simulink model "EXP4"  (R2020b)
settings: Solver=VariableStepAuto  StartTime=0.0  StopTime=0.02  RelTol=1e-3
libraries: powerlib x73, powerlib_meascontrol x2, simulink x2, simulink_extras x1
settings Model: Creator=pushp  LastModifiedBy=rupes
settings DebuggingCC: SFMachineParentedDataDiag=error  ArithmeticOperatorsInVariantConditions=warning
settings SFSimCC: CustomCodeUndefinedFunction=UseInterfaceOnly
settings CodeAppCC: StateflowObjectComments=on

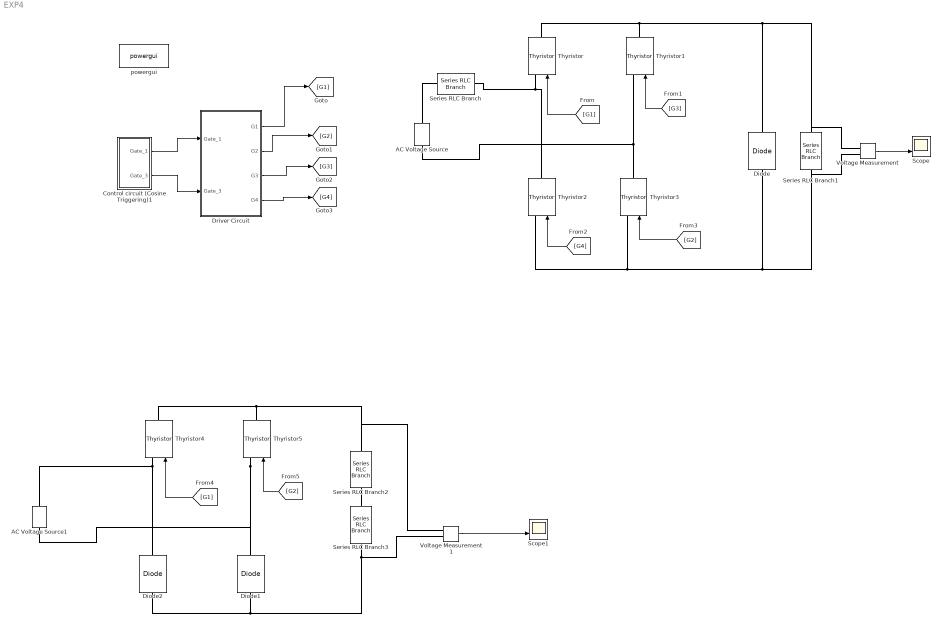
== system EXP4 ==
  AC Voltage Source : powerlib/Electrical Sources/AC Voltage Source  Amplitude=100  Phase=0  Frequency=60  SampleTime=0  Measurements=None  BusType=swing  Pref=10e3  Qref=0  Qmin=-inf  Qmax=+inf
  AC Voltage Source1 : powerlib/Electrical Sources/AC Voltage Source  Amplitude=100  Phase=0  Frequency=60  SampleTime=0  Measurements=None  BusType=swing  Pref=10e3  Qref=0  Qmin=-inf  Qmax=+inf
  Control circuit (Cosine Triggering)1 : Subsystem
  Diode : powerlib/Power Electronics/Diode  Ron=0.001  Lon=0  Vf=0.8  IC=0  UseSnubber=0  Rs=500  Cs=250e-9  Measurements=off
  Diode1 : powerlib/Power Electronics/Diode  Ron=0.001  Lon=0  Vf=0.8  IC=0  UseSnubber=0  Rs=500  Cs=250e-9  Measurements=off
  Diode2 : powerlib/Power Electronics/Diode  Ron=0.001  Lon=0  Vf=0.8  IC=0  UseSnubber=0  Rs=500  Cs=250e-9  Measurements=off
  Driver Circuit : Subsystem
  Scope : Scope  NumInputPorts=2
  Scope1 : Scope  NumInputPorts=2
  Series RLC Branch : powerlib/Elements/Series RLC Branch  LConnTagsString=__new0  RConnTagsString=__new0  BranchType=L  Resistance=1  Inductance=1e-3  SetiL0=off  InitialCurrent=0  Capacitance=1e-6  Setx0=off  InitialVoltage=0  Measurements=None
  Series RLC Branch1 : powerlib/Elements/Series RLC Branch  LConnTagsString=__new0  RConnTagsString=__new0  BranchType=R  Resistance=1  Inductance=1e-3  SetiL0=off  InitialCurrent=0  Capacitance=1e-6  Setx0=off  InitialVoltage=0  Measurements=None
  Series RLC Branch2 : powerlib/Elements/Series RLC Branch  LConnTagsString=__new0  RConnTagsString=__new0  BranchType=L  Resistance=1  Inductance=1e-3  SetiL0=off  InitialCurrent=0  Capacitance=1e-6  Setx0=off  InitialVoltage=0  Measurements=None
  Series RLC Branch3 : powerlib/Elements/Series RLC Branch  LConnTagsString=__new0  RConnTagsString=__new0  BranchType=R  Resistance=1  Inductance=1e-3  SetiL0=off  InitialCurrent=0  Capacitance=1e-6  Setx0=off  InitialVoltage=0  Measurements=None
  Thyristor{,1..5} (6 alike) : powerlib/Power Electronics/Thyristor  Ron=0.001  Lon=0  Vf=0.8  IC=0  Rs=500  Cs=250e-9  Measurements=off
  Voltage Measurement : powerlib/Measurements/Voltage Measurement  PhasorSimulation=off  OutputType=Complex  PSBequivalent=0
  Voltage Measurement1 : powerlib/Measurements/Voltage Measurement  PhasorSimulation=off  OutputType=Complex  PSBequivalent=0
  powergui : powerlib/powergui  Priority=1  SimulationMode=Discrete  SampleTime=1e-6  frequency=60  Iterations=50  frequencyindice=0  Pbase=100e6  ErrMax=1e-4  UnitsV=kV  UnitsW=MW  buscounter=0  FunctionMessages=off  echomessages=off  EnableUseOfTLC=off  CurrentSourceSwitches=off  DisableSnubberDevices=off  DisableRonSwitches=off  DisableVfSwitches=off  DisplayEquations=off  AutomaticDiscreteSolvers=off  SolverType=Tustin/Backward Euler (TBE)  Interpol=off  ExternalGateDelay=off  methode=off  Ts=100  x0status=blocks  SPID=on  SwTol=0  HookPort=off  NonlinearTolerance=1e-4  nMaxIteration=100  ContinueOnMaxIteration=off  RestoreLinks=warning  ResistiveCurrentMeasurement=off  Frange=[0:2:500]  Ylog=off  Xlog=on  ShowGrid=off  save=off  variable=ZData  structure=0  ZoomFFT=off  StartTime=0.0  cycles=1  DisplayStyle=1  fundamental=60  FreqAxis=off  MaxFrequency=1000  frequencyindicesteady=1  RmsSteady=1  display=off
  wires:
  Driver Circuit/4(G4) -> [G4]
  Driver Circuit/1(G1) -> [G1]
  Control circuit (Cosine Triggering)1/1(Gate_1) -> Driver Circuit/1(Gate_1)
  Control circuit (Cosine Triggering)1/2(Gate_3) -> Driver Circuit/2(Gate_3)
  Driver Circuit/3(G3) -> [G3]
  Driver Circuit/2(G2) -> [G2]
  [G1] -> Thyristor/1
  [G3] -> Thyristor1/1
  [G4] -> Thyristor2/1
  [G2] -> Thyristor3/1
  Voltage Measurement/1 -> Scope/2
  [G1] -> Thyristor4/1
  [G2] -> Thyristor5/1
  Voltage Measurement1/1 -> Scope1/2
  connections:
  Thyristor/LConn1 -- Series RLC Branch/RConn1 -- Thyristor2/RConn1
  AC Voltage Source/RConn1 -- Series RLC Branch/LConn1
  Diode/LConn1 -- Voltage Measurement/LConn2 -- Series RLC Branch1/RConn1 -- Thyristor3/LConn1 -- Thyristor2/LConn1
  Thyristor3/RConn1 -- AC Voltage Source/LConn1 -- Thyristor1/LConn1
  Thyristor1/RConn1 -- Thyristor/RConn1 -- Voltage Measurement/LConn1 -- Series RLC Branch1/LConn1 -- Diode/RConn1
  Thyristor5/RConn1 -- Voltage Measurement1/LConn1 -- Series RLC Branch2/LConn1 -- Thyristor4/RConn1
  Series RLC Branch3/RConn1 -- Diode1/LConn1 -- Diode2/LConn1 -- Voltage Measurement1/LConn2
  Thyristor5/LConn1 -- Diode1/RConn1 -- AC Voltage Source1/LConn1
  Thyristor4/LConn1 -- AC Voltage Source1/RConn1 -- Diode2/RConn1
  Series RLC Branch3/LConn1 -- Series RLC Branch2/RConn1

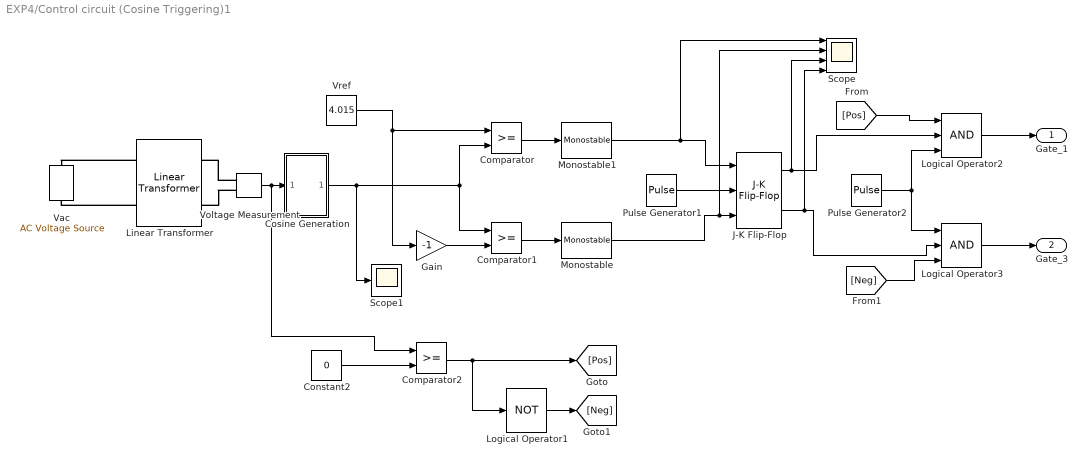
== system EXP4/Control circuit (Cosine Triggering)1 ==
  Comparator : RelationalOperator  OutDataTypeStr=boolean  RndMeth=Nearest
  Comparator1 : RelationalOperator  OutDataTypeStr=boolean  RndMeth=Nearest
  Comparator2 : RelationalOperator  OutDataTypeStr=boolean  RndMeth=Nearest
  Constant2 : Constant  Value=0
  Cosine Generation : Subsystem
  Gain : Gain  Gain=-1
  J-K Flip-Flop : simulink_extras/Flip Flops/J-K Flip-Flop  initial_condition=0
  Linear Transformer : powerlib/Elements/Linear Transformer  UNITS=pu  NominalPower=[4 50 ]  winding1=[230 6.9 7.1e-3 ]  winding2="[3.605 1.7e-3  2.1e-6]"  ThreeWindings=off  winding3=[ 315e3 0.002 0.08 ]  RmLm=[600 1.145]  Measurements=None  DataType=off
  Logical Operator1 : Logic  Operator=NOT  Inputs=inv  IconShape=distinctive  AllPortsSameDT=off  OutDataTypeStr=boolean
  Logical Operator2 : Logic  Inputs=3  IconShape=distinctive  AllPortsSameDT=off  OutDataTypeStr=boolean
  Logical Operator3 : Logic  Inputs=3  IconShape=distinctive  AllPortsSameDT=off  OutDataTypeStr=boolean
  Monostable : powerlib_meascontrol/Logic/Monostable  EdgeDetect=Rising  PulseDuration=1e-05  ic=0  Ts=0
      settings: SourceProductBaseCode=PS
  Monostable1 : powerlib_meascontrol/Logic/Monostable  EdgeDetect=Rising  PulseDuration=1e-05  ic=0  Ts=0
      settings: SourceProductBaseCode=PS
  Pulse Generator1 : DiscretePulseGenerator  PulseType=Time based  Period=2e-5  PulseWidth=50
  Pulse Generator2 : DiscretePulseGenerator  PulseType=Time based  Period=40e-6  PulseWidth=50
  Scope : Scope  NumInputPorts=4
  Scope1 : Scope
  Vac : powerlib/Electrical Sources/AC Voltage Source  Amplitude=230*sqrt(2)  Phase=0  Frequency=50  SampleTime=0  Measurements=None  BusType=swing  Pref=10e3  Qref=0  Qmin=-inf  Qmax=+inf
  Voltage Measurement : powerlib/Measurements/Voltage Measurement  PhasorSimulation=off  OutputType=Complex  PSBequivalent=0
  Vref : Constant  Value=4.015
  Gate_1 : Outport
  Gate_3 : Outport  Port=2
  wires:
  [Neg] -> Logical Operator3/3
  [Pos] -> Logical Operator2/1
  Logical Operator1/1 -> [Neg]
  Comparator2/1 -> [Pos], Logical Operator1/1
  Constant2/1 -> Comparator2/2
  Vref/1 -> Comparator/1, Gain/1
  Logical Operator3/1 -> Gate_3/1
  Logical Operator2/1 -> Gate_1/1
  Pulse Generator2/1 -> Logical Operator3/1, Logical Operator2/3
  J-K Flip-Flop/2 -> Scope/4, Logical Operator3/2
  J-K Flip-Flop/1 -> Logical Operator2/2, Scope/3
  Pulse Generator1/1 -> J-K Flip-Flop/2
  Monostable/1 -> Scope/2, J-K Flip-Flop/3
  Comparator1/1 -> Monostable/1
  Comparator/1 -> Monostable1/1
  Gain/1 -> Comparator1/2
  Cosine Generation/1(Out1) -> Scope1/1, Comparator/2, Comparator1/1
  Voltage Measurement/1 -> Cosine Generation/1(In1), Comparator2/1
  Monostable1/1 -> Scope/1, J-K Flip-Flop/1
  connections:
  Linear Transformer/LConn1 -- Vac/RConn1
  Linear Transformer/LConn2 -- Vac/LConn1
  Voltage Measurement/LConn1 -- Linear Transformer/RConn1
  Voltage Measurement/LConn2 -- Linear Transformer/RConn2

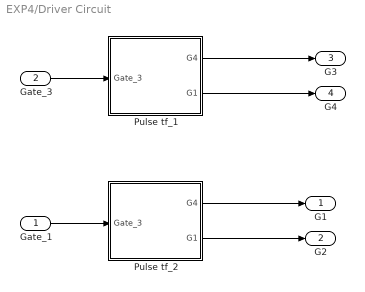
== system EXP4/Driver Circuit ==
  Gate_1 : Inport
  Gate_3 : Inport  Port=2
  Pulse tf_1 : Subsystem
  Pulse tf_2 : Subsystem
  G1 : Outport
  G2 : Outport  Port=2
  G3 : Outport  Port=3
  G4 : Outport  Port=4
  wires:
  Pulse tf_1/1(G4) -> G3/1
  Pulse tf_1/2(G1) -> G4/1
  Gate_3/1 -> Pulse tf_1/1(Gate_3)
  Gate_1/1 -> Pulse tf_2/1(Gate_3)
  Pulse tf_2/1(G4) -> G1/1
  Pulse tf_2/2(G1) -> G2/1

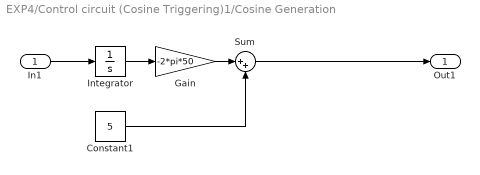
== system EXP4/Control circuit (Cosine Triggering)1/Cosine Generation ==
  In1 : Inport
  Constant1 : Constant  Value=5
  Gain : Gain  Gain=-2*pi*50
  Integrator : Integrator
  Sum : Sum  Inputs=|++
  Out1 : Outport
  wires:
  Sum/1 -> Out1/1
  Constant1/1 -> Sum/2
  In1/1 -> Integrator/1
  Integrator/1 -> Gain/1
  Gain/1 -> Sum/1

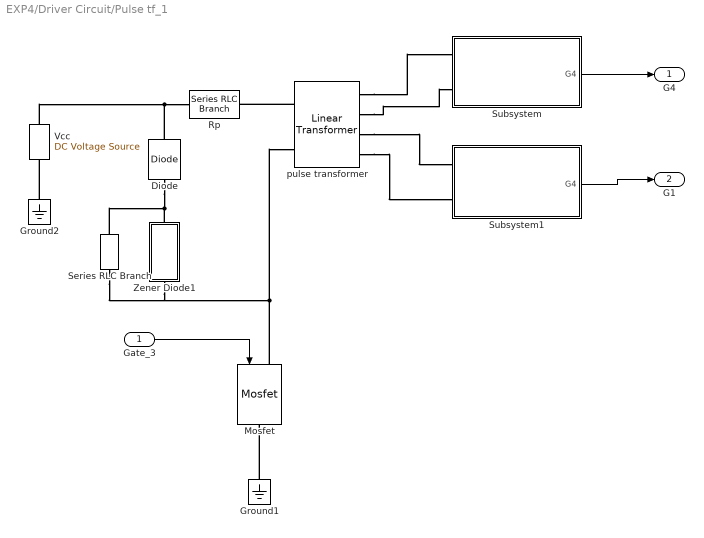
== system EXP4/Driver Circuit/Pulse tf_1 ==
  Gate_3 : Inport
  Diode : powerlib/Power Electronics/Diode  Ron=1  Lon=0  Vf=0.8  IC=0  UseSnubber=0  Rs=500  Cs=250e-9  Measurements=off
  Ground1 : powerlib/Elements/Ground  LConnTagsString=a
  Ground2 : powerlib/Elements/Ground  LConnTagsString=a
  Mosfet : powerlib/Power Electronics/Mosfet  Ron=0.1  Lon=0  Rd=0.01  Vfd=0  IC=0  Rs=1e5  Cs=inf  Measurements=off
  Rp : powerlib/Elements/Series RLC Branch  LConnTagsString=__new0  RConnTagsString=__new0  BranchType=R  Resistance=10  Inductance=1e-3  SetiL0=off  InitialCurrent=0  Capacitance=1e-6  Setx0=off  InitialVoltage=0  Measurements=None
  Series RLC Branch : powerlib/Elements/Series RLC Branch  LConnTagsString=__new0  RConnTagsString=__new0  BranchType=R  Resistance=1  Inductance=1e-3  SetiL0=off  InitialCurrent=0  Capacitance=1e-6  Setx0=off  InitialVoltage=0  Measurements=None
  Subsystem : Subsystem
  Subsystem1 : Subsystem
  Vcc : powerlib/Electrical Sources/DC Voltage Source  Amplitude=20  Measurements=None
  Zener Diode1 : Subsystem  mask(Zener Diode){Vz=10, Rzt=10, Rzk=400, Izm=400e-3, Vf=0.7, Ron=1e-3}
      mask prompts: Vz "Zener Voltage Vz (V)"; Rzt "Dynamic Impedance Zzt (ohms)"; Rzk "Knee Impedance Zzk (ohms)"; Izm "Maximum Continuous Current Izm (A)"; Vf "Forward Voltage Drop Vf (V)"; Ron "On Resistance Ron (ohms)"
      mask help:
      | Implements a zener diode block.
      | Use values from standard datasheets to populate block dialog
  pulse transformer : powerlib/Elements/Linear Transformer  UNITS=pu  NominalPower=[1 50e3 ]  winding1="[20  0.8 20e-6 ]"  winding2=[20 0.8 20e-6 ]  ThreeWindings=on  winding3=[20 0.8 20e-6]  RmLm=[ 400 1.5e-3 ]  Measurements=None  DataType=off
  G4 : Outport
  G1 : Outport  Port=2
  wires:
  Gate_3/1 -> Mosfet/1
  Subsystem1/1(G4) -> G1/1
  Subsystem/1(G4) -> G4/1
  connections:
  Zener Diode1/RConn1 -- Series RLC Branch/RConn1 -- pulse transformer/LConn2 -- Mosfet/LConn1
  Ground2/LConn1 -- Vcc/LConn1
  pulse transformer/LConn1 -- Rp/RConn1
  Series RLC Branch/LConn1 -- Zener Diode1/LConn1 -- Diode/LConn1
  Vcc/RConn1 -- Diode/RConn1 -- Rp/LConn1
  Ground1/LConn1 -- Mosfet/RConn1
  pulse transformer/RConn1 -- Subsystem/LConn1
  pulse transformer/RConn2 -- Subsystem/LConn2
  pulse transformer/RConn3 -- Subsystem1/LConn1
  pulse transformer/RConn4 -- Subsystem1/LConn2

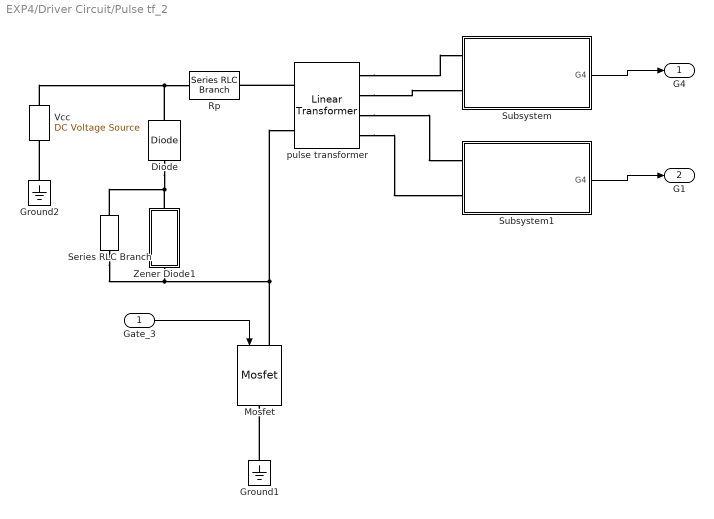
== system EXP4/Driver Circuit/Pulse tf_2 ==
  Gate_3 : Inport
  Diode : powerlib/Power Electronics/Diode  Ron=1  Lon=0  Vf=0.8  IC=0  UseSnubber=0  Rs=500  Cs=250e-9  Measurements=off
  Ground1 : powerlib/Elements/Ground  LConnTagsString=a
  Ground2 : powerlib/Elements/Ground  LConnTagsString=a
  Mosfet : powerlib/Power Electronics/Mosfet  Ron=0.1  Lon=0  Rd=0.01  Vfd=0  IC=0  Rs=1e5  Cs=inf  Measurements=off
  Rp : powerlib/Elements/Series RLC Branch  LConnTagsString=__new0  RConnTagsString=__new0  BranchType=R  Resistance=10  Inductance=1e-3  SetiL0=off  InitialCurrent=0  Capacitance=1e-6  Setx0=off  InitialVoltage=0  Measurements=None
  Series RLC Branch : powerlib/Elements/Series RLC Branch  LConnTagsString=__new0  RConnTagsString=__new0  BranchType=R  Resistance=1  Inductance=1e-3  SetiL0=off  InitialCurrent=0  Capacitance=1e-6  Setx0=off  InitialVoltage=0  Measurements=None
  Subsystem : Subsystem
  Subsystem1 : Subsystem
  Vcc : powerlib/Electrical Sources/DC Voltage Source  Amplitude=20  Measurements=None
  Zener Diode1 : Subsystem  mask(Zener Diode){Vz=10, Rzt=10, Rzk=400, Izm=400e-3, Vf=0.7, Ron=1e-3}
      mask prompts: Vz "Zener Voltage Vz (V)"; Rzt "Dynamic Impedance Zzt (ohms)"; Rzk "Knee Impedance Zzk (ohms)"; Izm "Maximum Continuous Current Izm (A)"; Vf "Forward Voltage Drop Vf (V)"; Ron "On Resistance Ron (ohms)"
      mask help:
      | Implements a zener diode block.
      | Use values from standard datasheets to populate block dialog
  pulse transformer : powerlib/Elements/Linear Transformer  UNITS=pu  NominalPower=[1 50e3]  winding1="[20  0.002  0.08 ]"  winding2="[20 0.002  0.08 ]"  ThreeWindings=on  winding3=[20 0.002 0.08 ]  RmLm=[400 1.5e-3 ]  Measurements=None  DataType=off
  G4 : Outport
  G1 : Outport  Port=2
  wires:
  Subsystem/1(G4) -> G4/1
  Subsystem1/1(G4) -> G1/1
  Gate_3/1 -> Mosfet/1
  connections:
  Vcc/RConn1 -- Diode/RConn1 -- Rp/LConn1
  Series RLC Branch/RConn1 -- Zener Diode1/RConn1 -- pulse transformer/LConn2 -- Mosfet/LConn1
  Series RLC Branch/LConn1 -- Zener Diode1/LConn1 -- Diode/LConn1
  Ground1/LConn1 -- Mosfet/RConn1
  pulse transformer/RConn1 -- Subsystem/LConn1
  pulse transformer/LConn1 -- Rp/RConn1
  Ground2/LConn1 -- Vcc/LConn1
  pulse transformer/RConn3 -- Subsystem1/LConn1
  pulse transformer/RConn4 -- Subsystem1/LConn2
  pulse transformer/RConn2 -- Subsystem/LConn2

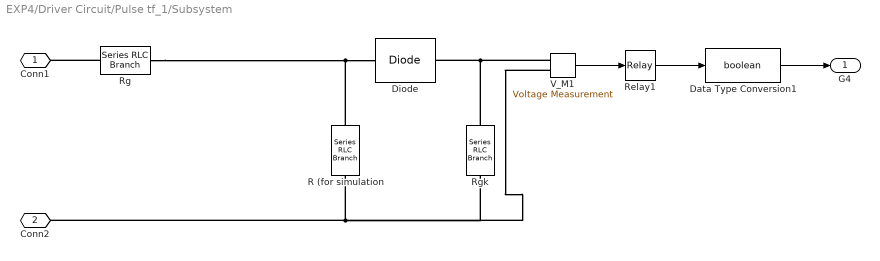
== system EXP4/Driver Circuit/Pulse tf_1/Subsystem ==
  Data Type Conversion1 : DataTypeConversion  OutDataTypeStr=boolean
  Diode : powerlib/Power Electronics/Diode  Ron=0.001  Lon=0  Vf=0.8  IC=0  UseSnubber=0  Rs=500  Cs=250e-9  Measurements=off
  R (for simulation : powerlib/Elements/Series RLC Branch  LConnTagsString=__new0  RConnTagsString=__new0  BranchType=R  Resistance=1  Inductance=1e-3  SetiL0=off  InitialCurrent=0  Capacitance=1e-6  Setx0=off  InitialVoltage=0  Measurements=None
  Relay1 : Relay  OnSwitchValue=0.36  OffSwitchValue=0.1
  Rg : powerlib/Elements/Series RLC Branch  LConnTagsString=__new0  RConnTagsString=__new0  BranchType=R  Resistance=20  Inductance=1e-3  SetiL0=off  InitialCurrent=0  Capacitance=1e-6  Setx0=off  InitialVoltage=0  Measurements=None
  Rgk : powerlib/Elements/Series RLC Branch  LConnTagsString=__new0  RConnTagsString=__new0  BranchType=R  Resistance=10  Inductance=1e-3  SetiL0=off  InitialCurrent=0  Capacitance=1e-6  Setx0=off  InitialVoltage=0  Measurements=None
  V_M1 : powerlib/Measurements/Voltage Measurement  PhasorSimulation=off  OutputType=Complex  PSBequivalent=0
  Conn1 : PMIOPort  Side=Left
  Conn2 : PMIOPort  Port=2  Side=Left
  G4 : Outport
  wires:
  Data Type Conversion1/1 -> G4/1
  Relay1/1 -> Data Type Conversion1/1
  V_M1/1 -> Relay1/1
  connections:
  V_M1/LConn2 -- Rgk/RConn1 -- R (for simulation/RConn1 -- Conn2/RConn1
  Rg/LConn1 -- Conn1/RConn1
  Rgk/LConn1 -- V_M1/LConn1 -- Diode/RConn1
  Rg/RConn1 -- Diode/LConn1 -- R (for simulation/LConn1

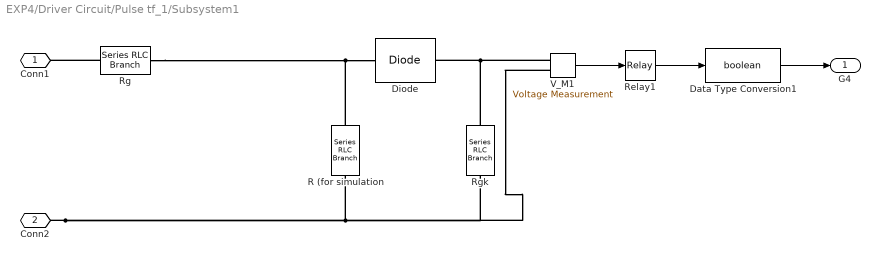
== system EXP4/Driver Circuit/Pulse tf_1/Subsystem1 ==
  Data Type Conversion1 : DataTypeConversion  OutDataTypeStr=boolean
  Diode : powerlib/Power Electronics/Diode  Ron=0.001  Lon=0  Vf=0.8  IC=0  UseSnubber=0  Rs=500  Cs=250e-9  Measurements=off
  R (for simulation : powerlib/Elements/Series RLC Branch  LConnTagsString=__new0  RConnTagsString=__new0  BranchType=R  Resistance=1  Inductance=1e-3  SetiL0=off  InitialCurrent=0  Capacitance=1e-6  Setx0=off  InitialVoltage=0  Measurements=None
  Relay1 : Relay  OnSwitchValue=0.36  OffSwitchValue=0.1
  Rg : powerlib/Elements/Series RLC Branch  LConnTagsString=__new0  RConnTagsString=__new0  BranchType=R  Resistance=20  Inductance=1e-3  SetiL0=off  InitialCurrent=0  Capacitance=1e-6  Setx0=off  InitialVoltage=0  Measurements=None
  Rgk : powerlib/Elements/Series RLC Branch  LConnTagsString=__new0  RConnTagsString=__new0  BranchType=R  Resistance=10  Inductance=1e-3  SetiL0=off  InitialCurrent=0  Capacitance=1e-6  Setx0=off  InitialVoltage=0  Measurements=None
  V_M1 : powerlib/Measurements/Voltage Measurement  PhasorSimulation=off  OutputType=Complex  PSBequivalent=0
  Conn1 : PMIOPort  Side=Left
  Conn2 : PMIOPort  Port=2  Side=Left
  G4 : Outport
  wires:
  Data Type Conversion1/1 -> G4/1
  Relay1/1 -> Data Type Conversion1/1
  V_M1/1 -> Relay1/1
  connections:
  Rgk/LConn1 -- V_M1/LConn1 -- Diode/RConn1
  Conn2/RConn1 -- R (for simulation/RConn1 -- V_M1/LConn2 -- Rgk/RConn1
  Rg/RConn1 -- Diode/LConn1 -- R (for simulation/LConn1
  Rg/LConn1 -- Conn1/RConn1

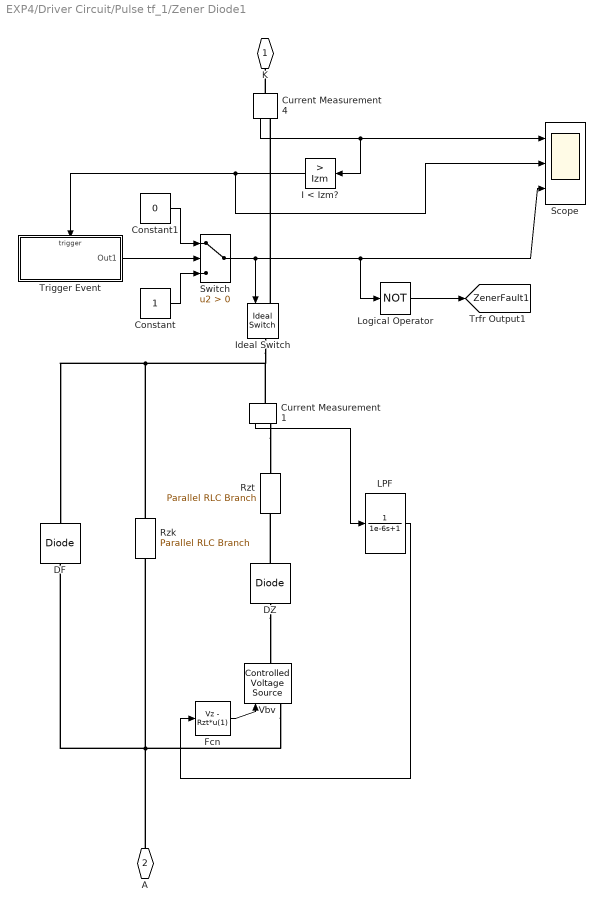
== system EXP4/Driver Circuit/Pulse tf_1/Zener Diode1 ==
  Constant : Constant
  Constant1 : Constant  Value=0
  Current Measurement1 : powerlib/Measurements/Current Measurement  PhasorSimulation=off  OutputType=Complex  PSBequivalent=0
  Current Measurement4 : powerlib/Measurements/Current Measurement  PhasorSimulation=off  OutputType=Complex  PSBequivalent=0
  DF : powerlib/Power Electronics/Diode  Ron=Ron  Lon=0  Vf=Vf  IC=0  UseSnubber=off  Rs=1000  Cs=0  Measurements=off
  DZ : powerlib/Power Electronics/Diode  Ron=1e-6  Lon=0  Vf=0  IC=0  UseSnubber=off  Rs=100  Cs=inf  Measurements=off
  Fcn : Fcn  Expr=Vz - Rzt*u(1)
  I < Izm? : simulink/Logic and Bit Operations/Compare To Constant  relop=>  const=Izm  OutDataTypeStr=boolean
  Ideal Switch : powerlib/Power Electronics/Ideal Switch  Ron=0.001  Lon=0  IC=1  Rs=1e5  Cs=0  Measurements=off
  LPF : TransferFcn  Denominator=[1e-6 1]
  Logical Operator : Logic  Operator=NOT  AllPortsSameDT=off  OutDataTypeStr=boolean
  Rzk : powerlib/Elements/Parallel RLC Branch  LConnTagsString=a  RConnTagsString=__new0  BranchType=R  Resistance=Rzk  Inductance=1.0  SetiL0=off  InitialCurrent=0  Capacitance=1e-5  Setx0=off  InitialVoltage=0  Measurements=None
  Rzt : powerlib/Elements/Parallel RLC Branch  LConnTagsString=a  RConnTagsString=__new0  BranchType=R  Resistance=Rzt  Inductance=1.0  SetiL0=off  InitialCurrent=0  Capacitance=1e-5  Setx0=off  InitialVoltage=0  Measurements=None
  Scope : Scope  NumInputPorts=3
  Switch : Switch  Criteria=u2 > Threshold
  Trigger Event : Subsystem  TreatAsAtomicUnit=on
  Vbv : powerlib/Electrical Sources/Controlled Voltage Source  Initialize=off  Source_Type=DC  Amplitude=0  Phase=0  Frequency=0  Measurements=None
  K : PMIOPort  Side=Left
  A : PMIOPort  Port=2  Side=Right
  tag scope: ZenerFault1=global
  wires:
  Fcn/1 -> Vbv/1
  Current Measurement4/1 -> Scope/1, I < Izm?/1
  Current Measurement1/1 -> LPF/1
  LPF/1 -> Fcn/1
  I < Izm?/1 -> Scope/2, Trigger Event/Trigger
  Switch/1 -> Ideal Switch/1, Scope/3, Logical Operator/1
  Trigger Event/1(Out1) -> Switch/2
  Constant/1 -> Switch/3
  Constant1/1 -> Switch/1
  Logical Operator/1 -> [ZenerFault1]
  connections:
  DZ/RConn1 -- Vbv/RConn1
  Current Measurement4/LConn1 -- K/RConn1
  DZ/LConn1 -- Rzt/LConn1
  Current Measurement1/RConn1 -- Rzt/RConn1
  Rzk/RConn1 -- Current Measurement1/LConn1 -- Ideal Switch/RConn1 -- DF/RConn1
  Ideal Switch/LConn1 -- Current Measurement4/RConn1
  A/RConn1 -- DF/LConn1 -- Rzk/LConn1 -- Vbv/LConn1

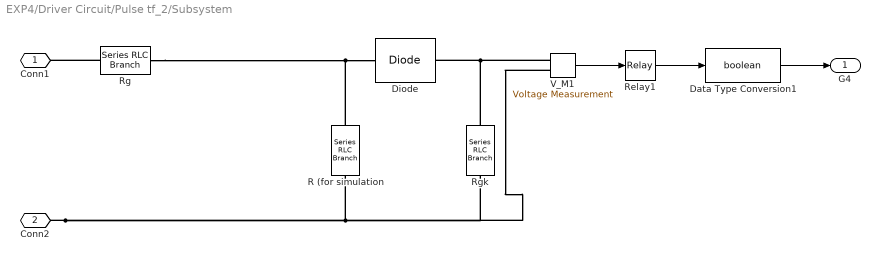
== system EXP4/Driver Circuit/Pulse tf_2/Subsystem ==
  Data Type Conversion1 : DataTypeConversion  OutDataTypeStr=boolean
  Diode : powerlib/Power Electronics/Diode  Ron=0.001  Lon=0  Vf=0.8  IC=0  UseSnubber=0  Rs=500  Cs=250e-9  Measurements=off
  R (for simulation : powerlib/Elements/Series RLC Branch  LConnTagsString=__new0  RConnTagsString=__new0  BranchType=R  Resistance=1  Inductance=1e-3  SetiL0=off  InitialCurrent=0  Capacitance=1e-6  Setx0=off  InitialVoltage=0  Measurements=None
  Relay1 : Relay  OnSwitchValue=0.36  OffSwitchValue=0.1
  Rg : powerlib/Elements/Series RLC Branch  LConnTagsString=__new0  RConnTagsString=__new0  BranchType=R  Resistance=20  Inductance=1e-3  SetiL0=off  InitialCurrent=0  Capacitance=1e-6  Setx0=off  InitialVoltage=0  Measurements=None
  Rgk : powerlib/Elements/Series RLC Branch  LConnTagsString=__new0  RConnTagsString=__new0  BranchType=R  Resistance=10  Inductance=1e-3  SetiL0=off  InitialCurrent=0  Capacitance=1e-6  Setx0=off  InitialVoltage=0  Measurements=None
  V_M1 : powerlib/Measurements/Voltage Measurement  PhasorSimulation=off  OutputType=Complex  PSBequivalent=0
  Conn1 : PMIOPort  Side=Left
  Conn2 : PMIOPort  Port=2  Side=Left
  G4 : Outport
  wires:
  Data Type Conversion1/1 -> G4/1
  Relay1/1 -> Data Type Conversion1/1
  V_M1/1 -> Relay1/1
  connections:
  Rgk/LConn1 -- V_M1/LConn1 -- Diode/RConn1
  Conn2/RConn1 -- R (for simulation/RConn1 -- V_M1/LConn2 -- Rgk/RConn1
  Rg/RConn1 -- Diode/LConn1 -- R (for simulation/LConn1
  Rg/LConn1 -- Conn1/RConn1

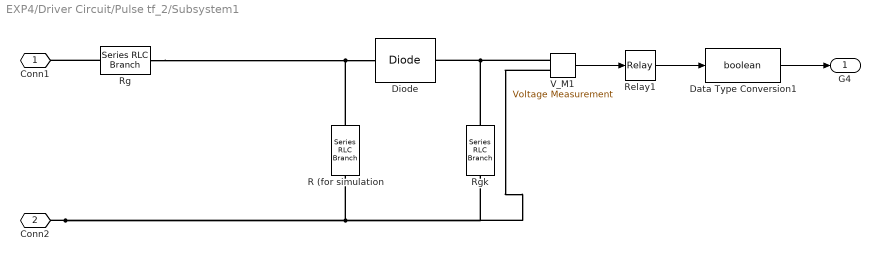
== system EXP4/Driver Circuit/Pulse tf_2/Subsystem1 ==
  Data Type Conversion1 : DataTypeConversion  OutDataTypeStr=boolean
  Diode : powerlib/Power Electronics/Diode  Ron=0.001  Lon=0  Vf=0.8  IC=0  UseSnubber=0  Rs=500  Cs=250e-9  Measurements=off
  R (for simulation : powerlib/Elements/Series RLC Branch  LConnTagsString=__new0  RConnTagsString=__new0  BranchType=R  Resistance=1  Inductance=1e-3  SetiL0=off  InitialCurrent=0  Capacitance=1e-6  Setx0=off  InitialVoltage=0  Measurements=None
  Relay1 : Relay  OnSwitchValue=0.36  OffSwitchValue=0.1
  Rg : powerlib/Elements/Series RLC Branch  LConnTagsString=__new0  RConnTagsString=__new0  BranchType=R  Resistance=20  Inductance=1e-3  SetiL0=off  InitialCurrent=0  Capacitance=1e-6  Setx0=off  InitialVoltage=0  Measurements=None
  Rgk : powerlib/Elements/Series RLC Branch  LConnTagsString=__new0  RConnTagsString=__new0  BranchType=R  Resistance=10  Inductance=1e-3  SetiL0=off  InitialCurrent=0  Capacitance=1e-6  Setx0=off  InitialVoltage=0  Measurements=None
  V_M1 : powerlib/Measurements/Voltage Measurement  PhasorSimulation=off  OutputType=Complex  PSBequivalent=0
  Conn1 : PMIOPort  Side=Left
  Conn2 : PMIOPort  Port=2  Side=Left
  G4 : Outport
  wires:
  Data Type Conversion1/1 -> G4/1
  Relay1/1 -> Data Type Conversion1/1
  V_M1/1 -> Relay1/1
  connections:
  Rgk/LConn1 -- V_M1/LConn1 -- Diode/RConn1
  Conn2/RConn1 -- R (for simulation/RConn1 -- V_M1/LConn2 -- Rgk/RConn1
  Rg/RConn1 -- Diode/LConn1 -- R (for simulation/LConn1
  Rg/LConn1 -- Conn1/RConn1

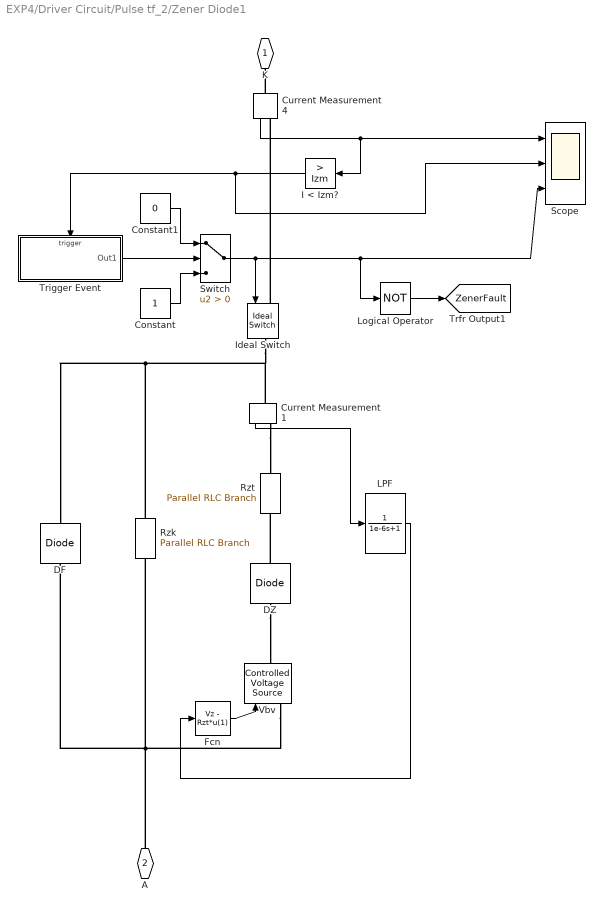
== system EXP4/Driver Circuit/Pulse tf_2/Zener Diode1 ==
  Constant : Constant
  Constant1 : Constant  Value=0
  Current Measurement1 : powerlib/Measurements/Current Measurement  PhasorSimulation=off  OutputType=Complex  PSBequivalent=0
  Current Measurement4 : powerlib/Measurements/Current Measurement  PhasorSimulation=off  OutputType=Complex  PSBequivalent=0
  DF : powerlib/Power Electronics/Diode  Ron=Ron  Lon=0  Vf=Vf  IC=0  UseSnubber=off  Rs=1000  Cs=0  Measurements=off
  DZ : powerlib/Power Electronics/Diode  Ron=1e-6  Lon=0  Vf=0  IC=0  UseSnubber=off  Rs=100  Cs=inf  Measurements=off
  Fcn : Fcn  Expr=Vz - Rzt*u(1)
  I < Izm? : simulink/Logic and Bit Operations/Compare To Constant  relop=>  const=Izm  OutDataTypeStr=boolean
  Ideal Switch : powerlib/Power Electronics/Ideal Switch  Ron=0.001  Lon=0  IC=1  Rs=1e5  Cs=0  Measurements=off
  LPF : TransferFcn  Denominator=[1e-6 1]
  Logical Operator : Logic  Operator=NOT  AllPortsSameDT=off  OutDataTypeStr=boolean
  Rzk : powerlib/Elements/Parallel RLC Branch  LConnTagsString=a  RConnTagsString=__new0  BranchType=R  Resistance=Rzk  Inductance=1.0  SetiL0=off  InitialCurrent=0  Capacitance=1e-5  Setx0=off  InitialVoltage=0  Measurements=None
  Rzt : powerlib/Elements/Parallel RLC Branch  LConnTagsString=a  RConnTagsString=__new0  BranchType=R  Resistance=Rzt  Inductance=1.0  SetiL0=off  InitialCurrent=0  Capacitance=1e-5  Setx0=off  InitialVoltage=0  Measurements=None
  Scope : Scope  NumInputPorts=3
  Switch : Switch  Criteria=u2 > Threshold
  Trigger Event : Subsystem  TreatAsAtomicUnit=on
  Vbv : powerlib/Electrical Sources/Controlled Voltage Source  Initialize=off  Source_Type=DC  Amplitude=0  Phase=0  Frequency=0  Measurements=None
  K : PMIOPort  Side=Left
  A : PMIOPort  Port=2  Side=Right
  tag scope: ZenerFault=global
  wires:
  Fcn/1 -> Vbv/1
  Current Measurement4/1 -> Scope/1, I < Izm?/1
  Current Measurement1/1 -> LPF/1
  LPF/1 -> Fcn/1
  I < Izm?/1 -> Scope/2, Trigger Event/Trigger
  Switch/1 -> Ideal Switch/1, Scope/3, Logical Operator/1
  Trigger Event/1(Out1) -> Switch/2
  Constant/1 -> Switch/3
  Constant1/1 -> Switch/1
  Logical Operator/1 -> [ZenerFault]
  connections:
  DZ/RConn1 -- Vbv/RConn1
  Current Measurement4/LConn1 -- K/RConn1
  DZ/LConn1 -- Rzt/LConn1
  Current Measurement1/RConn1 -- Rzt/RConn1
  Rzk/RConn1 -- Current Measurement1/LConn1 -- Ideal Switch/RConn1 -- DF/RConn1
  Ideal Switch/LConn1 -- Current Measurement4/RConn1
  A/RConn1 -- DF/LConn1 -- Rzk/LConn1 -- Vbv/LConn1

== system EXP4/Driver Circuit/Pulse tf_1/Zener Diode1/Trigger Event ==
  Trigger : TriggerPort  VariantControl=Variant  ShowOutputPort=on
  Scope2 : Scope
  Out1 : Outport  VectorParamsAs1DForOutWhenUnconnected=off
  wires:
  Trigger/1 -> Scope2/1, Out1/1

== system EXP4/Driver Circuit/Pulse tf_2/Zener Diode1/Trigger Event ==
  Trigger : TriggerPort  VariantControl=Variant  ShowOutputPort=on
  Scope2 : Scope
  Out1 : Outport  VectorParamsAs1DForOutWhenUnconnected=off
  wires:
  Trigger/1 -> Scope2/1, Out1/1
